simulink model "SIM4"  (R2023b)
settings: Solver=ode4  StartTime=0.0  StopTime=tf  FixedStep=dt  RelTol=1e-3
InitFcn:
  | I = diag([3,4,2]);
  | Iinv = inv(I);
  | 
  | dt = 0.01;
  | dtsim = 10;
  | 
  | q0 = [0;0;0;1];
  | w0 = [0.001;0.001;0.001];
  | 
  | mu = 398600; %km3/s2
  | H0 = 1e-4*[1;1;1];
  | r0 = [6678; 0; 0];
  | v0 = sqrt(mu/norm(r0)).*[0;1;0.2];
  | 
  | a = -mu/2/(norm(v0)^2/2 - mu/norm(r0));
  | tf = 2*pi*sqrt(a^3/mu);
  | 
  | myworld = vrworld('SpacecraftEarth.wrl');
  | 
  | open(myworld);
  | 
  | set(0,'Units','pixels');
  | 
  | scnsize = get(0,'ScreenSize');
  | 
  | f1 = vrfigure(myworld,[1 80 scnsize(3)/2 scnsize(4)/2]);
  | 
  | set(f1,'Viewpoint','WorldView')
  | 
  | f2 = vrfigure(myworld,[scnsize(3)/2 80 scnsize(3)/2 scnsize(4)/2]);
  | 
  | set(f2,'Viewpoint','TargetView')
libraries: vrlib x3, matrix_library x1
settings Model: Creator=David  LastModifiedBy=David

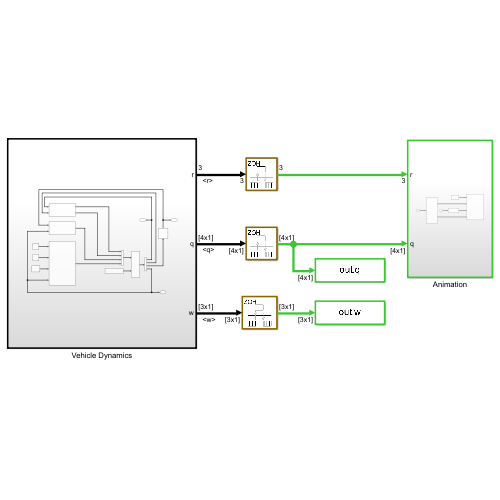
[thumbnail: Simulink's stored preview of the top-level diagram]
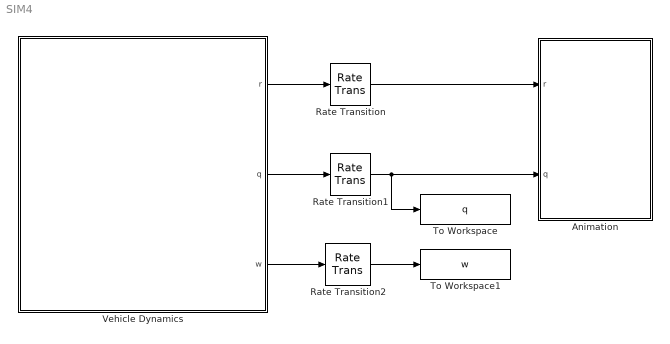
== system SIM4 ==
  Animation : Subsystem
  Rate Transition : RateTransition  InitialCondition=r0  OutPortSampleTime=dtsim
  Rate Transition1 : RateTransition  InitialCondition=q0  OutPortSampleTime=dtsim
  Rate Transition2 : RateTransition  InitialCondition=w0  OutPortSampleTime=dtsim
  To Workspace : ToWorkspace  VariableName=q  SampleTime=-1
  To Workspace1 : ToWorkspace  VariableName=w  SampleTime=-1
  Vehicle Dynamics : Subsystem
  wires:
  Vehicle Dynamics/1(r) -> Rate Transition/1
  Vehicle Dynamics/2(q) -> Rate Transition1/1
  Vehicle Dynamics/3(w) -> Rate Transition2/1
  Rate Transition/1 -> Animation/1(r)
  Rate Transition1/1 -> To Workspace/1, Animation/2(q)
  Rate Transition2/1 -> To Workspace1/1

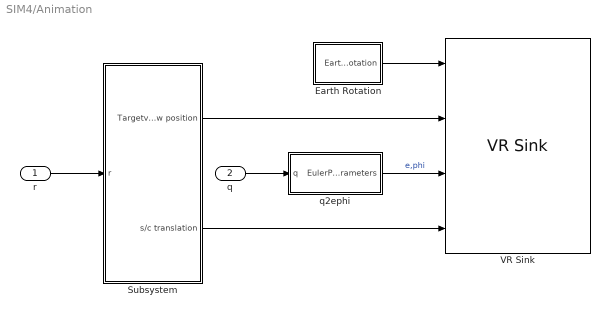
== system SIM4/Animation ==
  r : Inport
  q : Inport  Port=2
  Earth Rotation : Subsystem
  Subsystem : Subsystem
  VR Sink : vrlib/VR Sink  InstantiateOnLoad=on  SampleTime=dtsim  ViewEnable=on  RemoteChange=off  RemoteView=off  FieldsWritten=Earth.rotation.4.1.1.double#TargetView.position.3.1.1.double#Spacecraft.rotation.4.1.1.double#Spacecraft.translation.3.1.1.double  WorldFileName=SpacecraftEarth.wrl  WorldDescription=The Earth - Low Resolution Model  AutoView=off  VideoDimensions=[]  AllowVariableSize=off
  q2ephi : Subsystem
  wires:
  q/1 -> q2ephi/1(q)
  q2ephi/1(EulerParameters) -> VR Sink/3  "e,phi"
  Earth Rotation/1(Earth Rotation) -> VR Sink/1
  r/1 -> Subsystem/1(r)
  Subsystem/2(s/c translation) -> VR Sink/4
  Subsystem/1(Targetview position) -> VR Sink/2

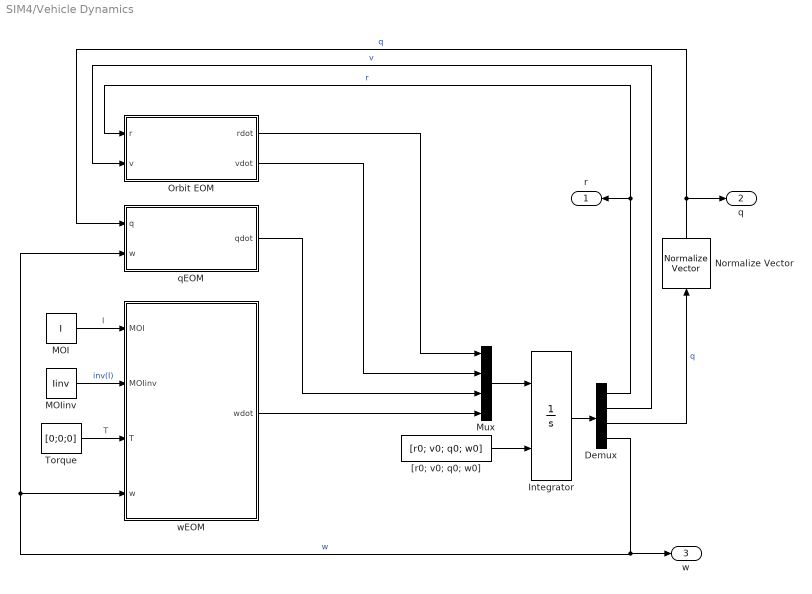
== system SIM4/Vehicle Dynamics ==
  Demux : Demux  Outputs=[3,3,4,3]
  Integrator : Integrator  InitialConditionSource=external
  MOI : Constant  Value=I
  MOIinv : Constant  Value=Iinv
  Mux : Mux
  Normalize Vector : vrlib/Utilities/Normalize Vector  maxzero=0
  Orbit EOM : Subsystem
  Torque : Constant  Value=[0;0;0]
  "[r0; v0; q0; w0]" : Constant  Value=[r0; v0; q0; w0]
  qEOM : Subsystem
  wEOM : Subsystem
  r : Outport
  q : Outport  Port=2
  w : Outport  Port=3
  wires:
  MOI/1 -> wEOM/1(MOI)  "I"
  Integrator/1 -> Demux/1
  qEOM/1(qdot) -> Mux/3
  Demux/4 -> w/1, qEOM/2(w), wEOM/4(w)  "w"
  "[r0; v0; q0; w0]"/1 -> Integrator/2
  Demux/3 -> Normalize Vector/1  "q"
  Torque/1 -> wEOM/3(T)  "T"
  wEOM/1(wdot) -> Mux/4
  Normalize Vector/1 -> qEOM/1(q), q/1  "q"
  MOIinv/1 -> wEOM/2(MOIinv)  "inv(I)"
  Mux/1 -> Integrator/1
  Orbit EOM/2(vdot) -> Mux/2
  Orbit EOM/1(rdot) -> Mux/1
  Demux/1 -> Orbit EOM/1(r), r/1  "r"
  Demux/2 -> Orbit EOM/2(v)  "v"

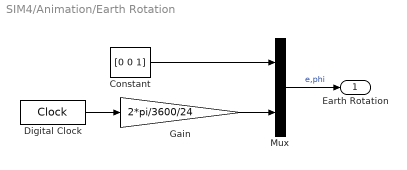
== system SIM4/Animation/Earth Rotation ==
  Constant : Constant  Value=[0 0 1]
  Digital Clock : DigitalClock  SampleTime=dtsim
  Gain : Gain  Gain=2*pi/3600/24
  Mux : Mux  Inputs=2
  Earth Rotation : Outport
  wires:
  Digital Clock/1 -> Gain/1
  Gain/1 -> Mux/2
  Mux/1 -> Earth Rotation/1  "e,phi"
  Constant/1 -> Mux/1

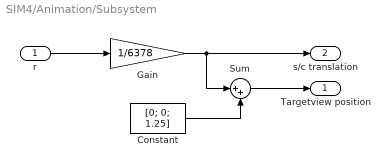
== system SIM4/Animation/Subsystem ==
  r : Inport
  Constant : Constant  Value=[0; 0; 1.25]
  Gain : Gain  Gain=1/6378
  Sum : Sum  Inputs=|++
  Targetview position : Outport
  s/c translation : Outport  Port=2
  wires:
  r/1 -> Gain/1
  Gain/1 -> s/c translation/1, Sum/1
  Sum/1 -> Targetview position/1
  Constant/1 -> Sum/2

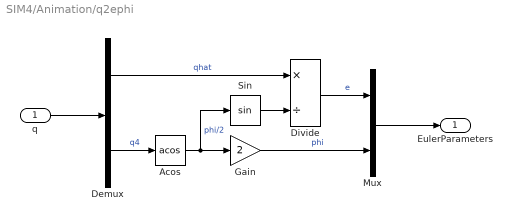
== system SIM4/Animation/q2ephi ==
  q : Inport  PortDimensions=[4;1]
  Acos : Trigonometry  Operator=acos
  Demux : Demux  Outputs=[3,1]
  Divide : Product  Inputs=*/
  Gain : Gain  Gain=2
  Mux : Mux  Inputs=2
  Sin : Trigonometry
  EulerParameters : Outport
  wires:
  q/1 -> Demux/1
  Acos/1 -> Gain/1, Sin/1  "phi/2"
  Sin/1 -> Divide/2
  Demux/1 -> Divide/1  "qhat"
  Demux/2 -> Acos/1  "q4"
  Divide/1 -> Mux/1  "e"
  Gain/1 -> Mux/2  "phi"
  Mux/1 -> EulerParameters/1

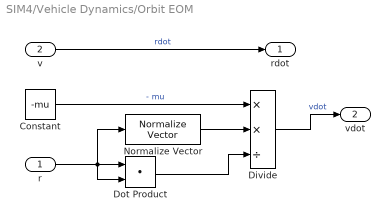
== system SIM4/Vehicle Dynamics/Orbit EOM ==
  r : Inport  PortDimensions=[3 1]
  v : Inport  Port=2
  Constant : Constant  Value=-mu
  Divide : Product  Inputs=**/
  Dot Product : DotProduct  OutDataTypeStr=Inherit: Inherit via internal rule
  Normalize Vector : vrlib/Utilities/Normalize Vector  maxzero=0
  rdot : Outport
  vdot : Outport  Port=2
  wires:
  v/1 -> rdot/1  "rdot"
  Constant/1 -> Divide/1  "- mu"
  Divide/1 -> vdot/1  "vdot"
  r/1 -> Dot Product/2, Dot Product/1, Normalize Vector/1
  Normalize Vector/1 -> Divide/2
  Dot Product/1 -> Divide/3

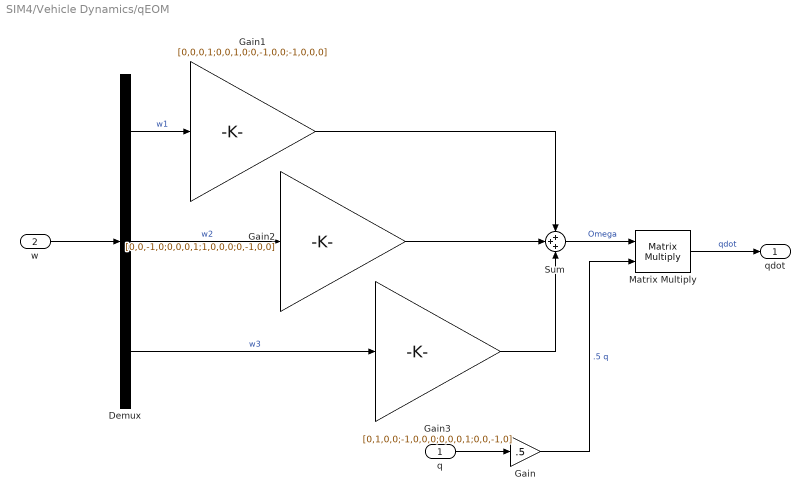
== system SIM4/Vehicle Dynamics/qEOM ==
  q : Inport
  w : Inport  Port=2
  Demux : Demux  Outputs=3
  Gain : Gain  Gain=.5
  Gain1 : Gain  Gain=[0,0,0,1;0,0,1,0;0,-1,0,0;-1,0,0,0]
  Gain2 : Gain  Gain=[0,0,-1,0;0,0,0,1;1,0,0,0;0,-1,0,0]
  Gain3 : Gain  Gain=[0,1,0,0;-1,0,0,0;0,0,0,1;0,0,-1,0]
  Matrix Multiply : Product  Multiplication=Matrix(*)
  Sum : Sum  Inputs=+++
  qdot : Outport
  wires:
  q/1 -> Gain/1
  Matrix Multiply/1 -> qdot/1  "qdot"
  Gain/1 -> Matrix Multiply/2  ".5 q"
  w/1 -> Demux/1
  Demux/1 -> Gain1/1  "w1"
  Demux/2 -> Gain2/1  "w2"
  Demux/3 -> Gain3/1  "w3"
  Gain2/1 -> Sum/2
  Gain3/1 -> Sum/3
  Gain1/1 -> Sum/1
  Sum/1 -> Matrix Multiply/1  "Omega"

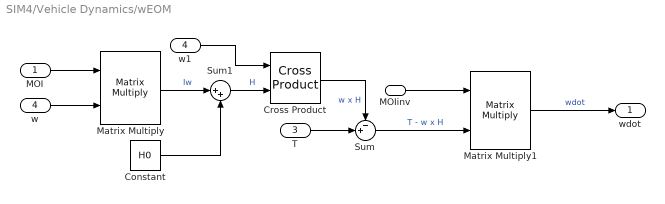
== system SIM4/Vehicle Dynamics/wEOM ==
  MOI : Inport
  MOIinv : Inport  Port=2
  T : Inport  Port=3
  w : Inport  Port=4
  Constant : Constant  Value=H0
  Cross Product : matrix_library/Cross Product
  Matrix Multiply : Product  Multiplication=Matrix(*)
  Matrix Multiply1 : Product  Multiplication=Matrix(*)
  Sum : Sum  Inputs=-+|
  Sum1 : Sum  Inputs=|++
  w1 : InportShadow  Port=4
  wdot : Outport
  wires:
  T/1 -> Sum/2
  MOI/1 -> Matrix Multiply/1
  w/1 -> Matrix Multiply/2
  w1/1 -> Cross Product/1
  Cross Product/1 -> Sum/1  "w x H"
  MOIinv/1 -> Matrix Multiply1/1
  Sum/1 -> Matrix Multiply1/2  "T - w x H"
  Matrix Multiply1/1 -> wdot/1  "wdot"
  Constant/1 -> Sum1/2
  Matrix Multiply/1 -> Sum1/1  "Iw"
  Sum1/1 -> Cross Product/2  "H"
